simulink model "LQR"  (R2024b)
settings: Solver=ode45  StartTime=0.0  StopTime=10.0  FixedStep=0.01  MaxStep=0.01  RelTol=1e-3
values from neighbouring files (symbols this model uses):
  d1 = 0.01    [Data_file_LQR.m]    (also in Data_file_LQR_Large_Force.m; Data_file_LQR_constant_force.m; Data_file_LQR_zero_force.m)
  d2 = 0.01    [Data_file_LQR.m]    (also in Data_file_LQR_Large_Force.m; Data_file_LQR_constant_force.m; Data_file_LQR_zero_force.m)
  F = 100    [Data_file_LQR.m]    (also in Data_file_LQR_Large_Force.m = 50; Data_file_LQR_constant_force.m = 10; Data_file_LQR_zero_force.m = 0)
  g = 9.81    [Data_file_LQR.m]    (also in Data_file_LQR_Large_Force.m; Data_file_LQR_constant_force.m; Data_file_LQR_zero_force.m)
  g_q = [1;0]    [Data_file_LQR.m]    (also in Data_file_LQR_Large_Force.m; Data_file_LQR_constant_force.m; Data_file_LQR_zero_force.m = [1; 0])
  K_lqr = [-14.1421000000000,171.884600000000,-25.2787000000000,54.7535000000000]    [Data_file_LQR.m]    (also in Data_file_LQR_Large_Force.m; Data_file_LQR_constant_force.m; Data_file_LQR_zero_force.m = [-14.1421000000000, 171.884600000000, -25.2787000000000, 54.)
  L = 1    [Data_file_LQR.m]    (also in Data_file_LQR_Large_Force.m; Data_file_LQR_constant_force.m; Data_file_LQR_zero_force.m)
  mc = 1.5    [Data_file_LQR.m]    (also in Data_file_LQR_Large_Force.m; Data_file_LQR_constant_force.m; Data_file_LQR_zero_force.m)
  mp = 0.5    [Data_file_LQR.m]    (also in Data_file_LQR_Large_Force.m; Data_file_LQR_constant_force.m; Data_file_LQR_zero_force.m)
  x_0 = [0.100000000000000;0.174532925199433;0;0]    [Data_file_LQR.m]    (also in Data_file_LQR_Large_Force.m; Data_file_LQR_constant_force.m; Data_file_LQR_zero_force.m = [0.100000000000000; 0.174532925199433; 0; 0])
settings Model: Creator=AA  LastModifiedBy=Marco
settings SolverCC: AlgebraicLoopSolver=TrustRegion
settings DataIOCC: ReturnWorkspaceOutputs=off  Refine=20
settings DebuggingCC: UnconnectedInputMsg=warning  UnconnectedOutputMsg=warning  UnconnectedLineMsg=warning  ArithmeticOperatorsInVariantConditions=warning
settings ModelReferenceCC: EnableRefExpFcnMdlSchedulingChecks=on
settings SFSimCC: SimUseLocalCustomCode=off  CustomCodeUndefinedFunction=UseInterfaceOnly
settings RTWCC: RTWUseLocalCustomCode=off  GPUComputeCapability=3.5

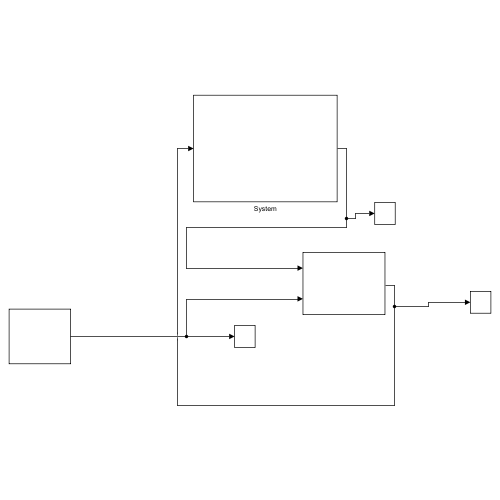
[thumbnail: Simulink's stored preview of the top-level diagram]
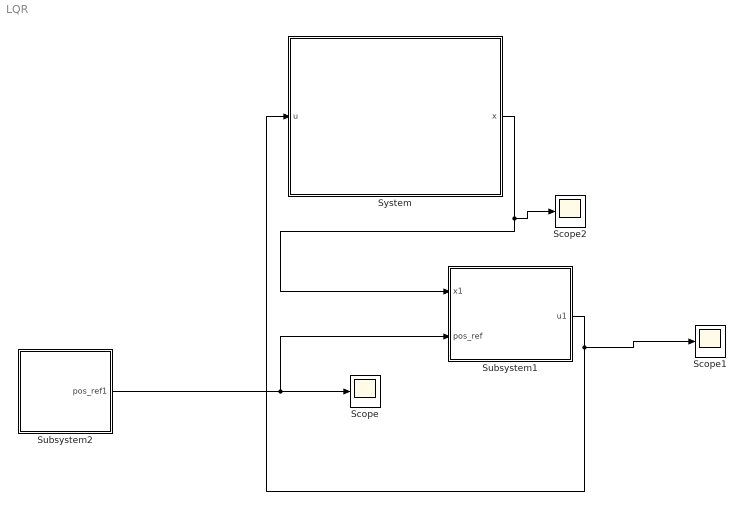
== system LQR ==
  Scope : Scope
  Scope1 : Scope
  Scope2 : Scope
  Subsystem1 : Subsystem
  Subsystem2 : Subsystem
  System : Subsystem
  wires:
  System/1(x) -> Scope2/1, Subsystem1/1(x1)
  Subsystem2/1(pos_ref1) -> Scope/1, Subsystem1/2(pos_ref)
  Subsystem1/1(u1) -> Scope1/1, System/1(u)

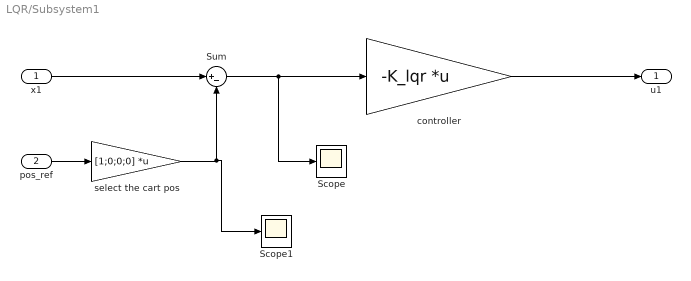
== system LQR/Subsystem1 ==
  x1 : Inport
  pos_ref : Inport  Port=2
  Scope : Scope
  Scope1 : Scope
  Sum : Sum  Inputs=|+-
  controller : Gain  Gain=-K_lqr  Multiplication=Matrix(K*u)
  select the cart pos : Gain  Gain=[1;0;0;0]  Multiplication=Matrix(K*u)
  u1 : Outport  VectorParamsAs1DForOutWhenUnconnected=off
  wires:
  x1/1 -> Sum/1
  pos_ref/1 -> select the cart pos/1
  Sum/1 -> Scope/1, controller/1
  controller/1 -> u1/1
  select the cart pos/1 -> Scope1/1, Sum/2

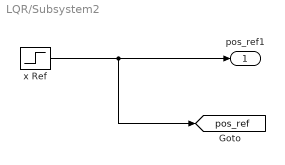
== system LQR/Subsystem2 ==
  x Ref : Step  After=3  SampleTime=0
  pos_ref1 : Outport  VectorParamsAs1DForOutWhenUnconnected=off
  tag scope: pos_ref=global
  wires:
  x Ref/1 -> pos_ref1/1, [pos_ref]

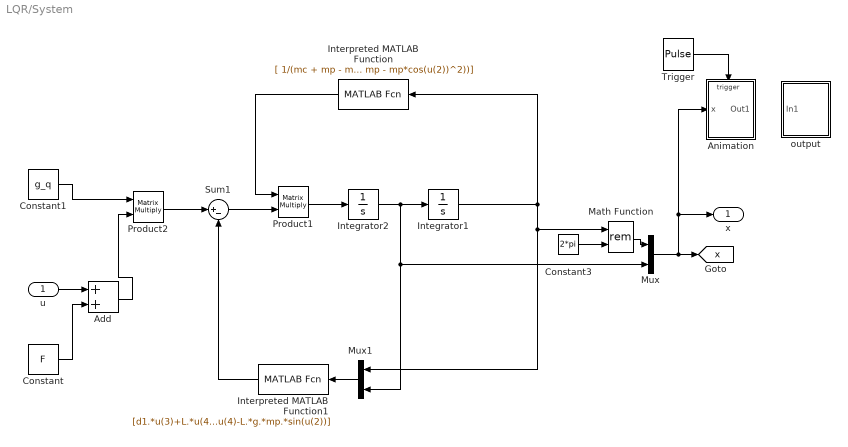
== system LQR/System ==
  u : Inport
  Add : Sum
  Animation : Subsystem
  Constant : Constant  Value=F
  Constant1 : Constant  Value=g_q
  Constant3 : Constant  Value=2*pi
  Integrator1 : Integrator  InitialCondition=x_0(1:2)
  Integrator2 : Integrator  InitialCondition=x_0(3:4)
  Interpreted MATLAB Function : MATLABFcn  MATLABFcn="[ 1/(mc + mp - mp*cos(u(2))^2),        cos(u(2))/(L*(mc + mp - mp*cos(u(2))^2)); cos(u(2))/(L*(mc + mp - mp*cos(u(2))^2)), (mc + mp)/(L^2*mp*(mc + mp - mp*cos(u(2))^2))]"  Output1D=off
  Interpreted MATLAB Function1 : MATLABFcn  MATLABFcn=[d1.*u(3)+L.*u(4).^2.*mp.*sin(u(2));d2.*u(4)-L.*g.*mp.*sin(u(2))]
  Math Function : Math  Operator=rem  SignedPower=on
  Mux : Mux  Inputs=2
  Mux1 : Mux  Inputs=2
  Product1 : Product  Multiplication=Matrix(*)
  Product2 : Product  Multiplication=Matrix(*)
  Sum1 : Sum  Inputs=|+-
  Trigger : DiscretePulseGenerator  PulseType=Time based  Period=0.1  PulseWidth=50
  output : Subsystem
  x : Outport  VectorParamsAs1DForOutWhenUnconnected=off
  tag scope: x=global
  wires:
  Mux/1 -> x/1, Animation/1(x), [x]
  Integrator2/1 -> Mux1/2, Mux/2, Integrator1/1
  Interpreted MATLAB Function/1 -> Product1/1
  Interpreted MATLAB Function1/1 -> Sum1/2
  Product1/1 -> Integrator2/1
  Constant3/1 -> Math Function/2
  Math Function/1 -> Mux/1
  Sum1/1 -> Product1/2
  Trigger/1 -> Animation/Trigger
  Integrator1/1 -> Interpreted MATLAB Function/1, Mux1/1, Math Function/1
  Constant1/1 -> Product2/1
  Mux1/1 -> Interpreted MATLAB Function1/1
  Product2/1 -> Sum1/1
  u/1 -> Add/1
  Constant/1 -> Add/2
  Add/1 -> Product2/2

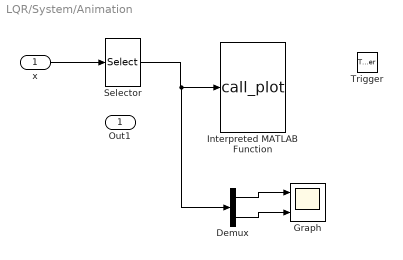
== system LQR/System/Animation ==
  x : Inport
  Trigger : TriggerPort  VariantControl=(inherit)  PortDimensions=1
  Demux : Demux  Outputs=2
  Graph : Scope  NumInputPorts=2
  Interpreted MATLAB Function : MATLABFcn  MATLABFcn=call_plot  OutputDimensions=0
  Selector : Selector  InputPortWidth=4  IndexOptions=Index vector (dialog)  Indices=[1:2]  OutputSizes=1
  Out1 : Outport
  wires:
  x/1 -> Selector/1
  Selector/1 -> Demux/1, Interpreted MATLAB Function/1
  Demux/1 -> Graph/1
  Demux/2 -> Graph/2

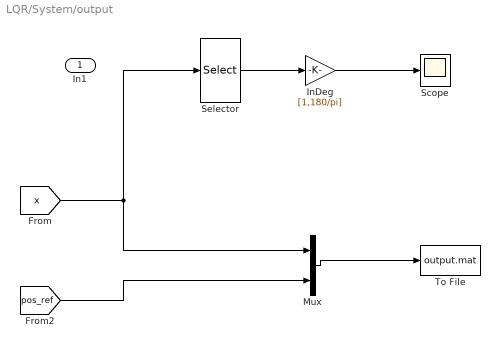
== system LQR/System/output ==
  In1 : Inport
  InDeg : Gain  Gain=[1,180/pi]
  Mux : Mux  Inputs=2
  Scope : Scope
  Selector : Selector  InputPortWidth=4  IndexOptions=Index vector (dialog)  Indices=[1:2]  OutputSizes=1
  To File : ToFile  Filename=output.mat  MatrixName=out  SaveFormat=Timeseries
  wires:
  [x] -> Mux/1, Selector/1
  InDeg/1 -> Scope/1
  Selector/1 -> InDeg/1
  Mux/1 -> To File/1
  [pos_ref] -> Mux/2
